simulink model "THREE_PID"  (R2019b)
settings: Solver=FixedStepAuto  StartTime=0.0  StopTime=20.0  FixedStep=1e-3  RelTol=1e-4
values from neighbouring files (symbols this model uses):
  D1 = P_kr/COEF_D1    (= 0.4625)    [code6.m]
  D2 = P_kr/COEF_D2    (= 1.23333333333)    [code6.m]
  D3 = P_kr/COEF_D3    (= 1.23333333333)    [code6.m]
  I1 = P_kr/COEF_I1    (= 1.85)    [code6.m]
  I2 = P_kr/COEF_I2    (= 1.85)    [code6.m]
  I3 = P_kr/COEF_I3    (= 1.85)    [code6.m]
  P1 = COEF_P1*K_kr    [code6.m]
  P2 = COEF_P2*K_kr    [code6.m]
  P3 = COEF_P3*K_kr    [code6.m]
settings Model: Creator=Szymon  LastModifiedBy=Szymon

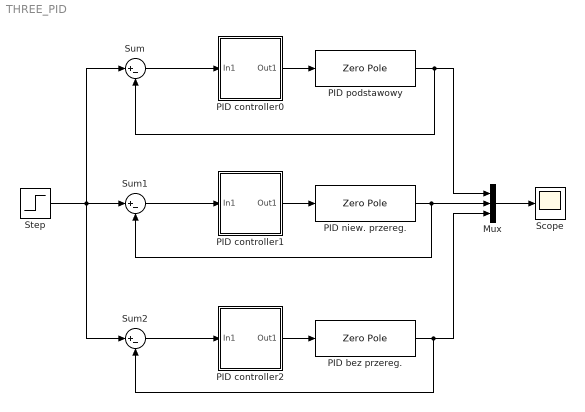
== system THREE_PID ==
  Mux : Mux  Inputs=3
  PID bez przereg. : ZeroPole  Zeros=[]  Poles=[-1 -1 -1]
  PID controller0 : Subsystem  mask{P=P1, I=I1, D=D1}
  PID controller1 : Subsystem  mask{P=P2, I=I2, D=D2}
  PID controller2 : Subsystem  mask{P=P3, I=I3, D=D3}
  PID niew. przereg. : ZeroPole  Zeros=[]  Poles=[-1 -1 -1]
  PID podstawowy : ZeroPole  Zeros=[]  Poles=[-1 -1 -1]
  Scope : Scope
  Step : Step  SampleTime=0
  Sum : Sum  Inputs=|+-
  Sum1 : Sum  Inputs=|+-
  Sum2 : Sum  Inputs=|+-
  wires:
  PID bez przereg./1 -> Sum2/2, Mux/3
  PID controller2/1(Out1) -> PID bez przereg./1
  PID controller0/1(Out1) -> PID podstawowy/1
  Step/1 -> Sum2/1, Sum/1, Sum1/1
  Sum2/1 -> PID controller2/1(In1)
  PID controller1/1(Out1) -> PID niew. przereg./1
  Sum/1 -> PID controller0/1(In1)
  PID niew. przereg./1 -> Sum1/2, Mux/2
  PID podstawowy/1 -> Sum/2, Mux/1
  Sum1/1 -> PID controller1/1(In1)
  Mux/1 -> Scope/1

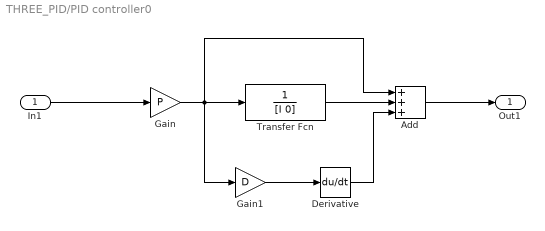
== system THREE_PID/PID controller0 ==
  In1 : Inport
  Add : Sum  Inputs=+++
  Derivative : Derivative
  Gain : Gain  Gain=P
  Gain1 : Gain  Gain=D
  Transfer Fcn : TransferFcn  Denominator=[I 0]
  Out1 : Outport
  wires:
  Gain1/1 -> Derivative/1
  Derivative/1 -> Add/3
  Gain/1 -> Add/1, Gain1/1, Transfer Fcn/1
  Add/1 -> Out1/1
  Transfer Fcn/1 -> Add/2
  In1/1 -> Gain/1

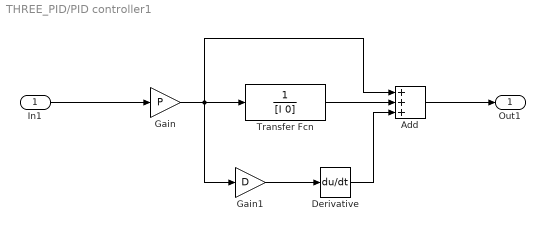
== system THREE_PID/PID controller1 ==
  In1 : Inport
  Add : Sum  Inputs=+++
  Derivative : Derivative
  Gain : Gain  Gain=P
  Gain1 : Gain  Gain=D
  Transfer Fcn : TransferFcn  Denominator=[I 0]
  Out1 : Outport
  wires:
  Gain1/1 -> Derivative/1
  Derivative/1 -> Add/3
  Gain/1 -> Add/1, Gain1/1, Transfer Fcn/1
  Add/1 -> Out1/1
  Transfer Fcn/1 -> Add/2
  In1/1 -> Gain/1

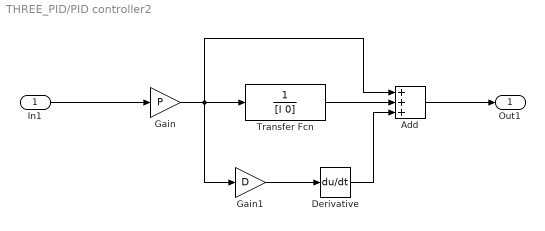
== system THREE_PID/PID controller2 ==
  In1 : Inport
  Add : Sum  Inputs=+++
  Derivative : Derivative
  Gain : Gain  Gain=P
  Gain1 : Gain  Gain=D
  Transfer Fcn : TransferFcn  Denominator=[I 0]
  Out1 : Outport
  wires:
  Gain1/1 -> Derivative/1
  Derivative/1 -> Add/3
  Gain/1 -> Add/1, Gain1/1, Transfer Fcn/1
  Add/1 -> Out1/1
  Transfer Fcn/1 -> Add/2
  In1/1 -> Gain/1
